simulink model "Bai2_TricycleDrive"  (R2018a)
settings: Solver=VariableStepAuto  StartTime=0.0  StopTime=200  RelTol=1e-3
libraries: simulink x1
settings Model: Creator=Administrator  LastModifiedBy=Administrator

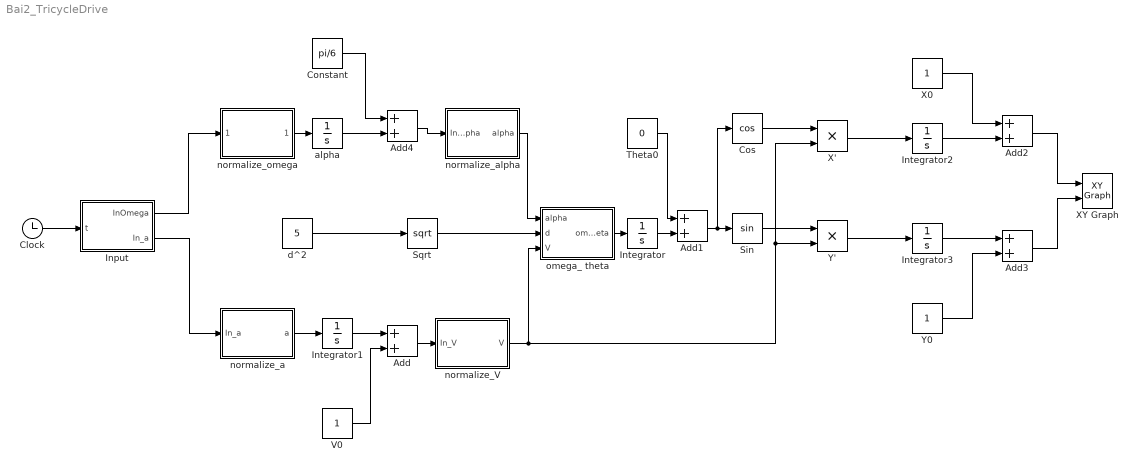
== system Bai2_TricycleDrive ==
  Add{,1..4} (5 alike) : Sum
  Clock : Clock
  Constant : Constant  Value=pi/6
  Cos : Trigonometry  Operator=cos
  Input : MATLAB Function  TreatAsAtomicUnit=on
  Integrator{,1..3} (4 alike) : Integrator
  Sin : Trigonometry
  Sqrt : Sqrt  SaturateOnIntegerOverflow=on
  Theta0 : Constant  Value=0
  V0 : Constant
  X' : Product
  X0 : Constant
  XY Graph : simulink/Sinks/XY Graph  xmin=-10  xmax=10  ymin=0  ymax=20  st=-1
  Y' : Product
  Y0 : Constant
  alpha : Integrator
  d^2 : Constant  Value=5
  normalize_V : MATLAB Function  TreatAsAtomicUnit=on
  normalize_a : MATLAB Function  TreatAsAtomicUnit=on
  normalize_alpha : MATLAB Function  TreatAsAtomicUnit=on
  normalize_omega : MATLAB Function  TreatAsAtomicUnit=on
  omega_ theta : MATLAB Function  TreatAsAtomicUnit=on
  wires:
  Clock/1 -> Input/1(t)
  Input/1(InOmega) -> normalize_omega/1(InOmega)
  Input/2(In_a) -> normalize_a/1(In_a)
  normalize_omega/1(Omega) -> alpha/1
  Add1/1 -> Cos/1, Sin/1
  normalize_a/1(a) -> Integrator1/1
  Integrator1/1 -> Add/1
  Sin/1 -> Y'/1
  Cos/1 -> X'/1
  normalize_V/1(V) -> omega_ theta/3(V), Y'/2, X'/2
  Add/1 -> normalize_V/1(In_V)
  V0/1 -> Add/2
  Theta0/1 -> Add1/1
  X'/1 -> Integrator2/1
  Y'/1 -> Integrator3/1
  Y0/1 -> Add3/2
  Integrator3/1 -> Add3/1
  X0/1 -> Add2/1
  Integrator2/1 -> Add2/2
  Add2/1 -> XY Graph/1
  Add3/1 -> XY Graph/2
  d^2/1 -> Sqrt/1
  Sqrt/1 -> omega_ theta/2(d)
  normalize_alpha/1(alpha) -> omega_ theta/1(alpha)
  Integrator/1 -> Add1/2
  omega_ theta/1(omega_theta) -> Integrator/1
  alpha/1 -> Add4/2
  Add4/1 -> normalize_alpha/1(In_alpha)
  Constant/1 -> Add4/1

== matlab function Bai2_TricycleDrive/normalize_omega ==
  data: InOmega input; Omega output
function Omega = fcn(InOmega)

if(InOmega >= 0.3) Omega = 0.3;
elseif(InOmega <= -0.3) Omega = -0.3;
else Omega = InOmega;
end

== matlab function Bai2_TricycleDrive/Input ==
  data: InOmega output; t input; In_a output
function [InOmega, In_a]= fcn(t)

% a) Van toc va goc lai khong doi
InOmega = 0;
In_a = 0;

% b) Van toc co dinh va goc lai thay doi theo thoi gian
%InOmega = 0.05;
%In_a = 0;

% c) Van toc va goc lai co dinh theo thoi gian
%InOmega = 0.05;
%In_a = 0.1;

== matlab function Bai2_TricycleDrive/normalize_alpha ==
  data: In_alpha input; alpha output
function alpha = fcn(In_alpha)

if(In_alpha >= 3.14/4) alpha = 3.14/4;
elseif(In_alpha <= -3.14/4) alpha = -3.14/4;
else alpha = In_alpha;
end

== matlab function Bai2_TricycleDrive/normalize_a ==
  data: In_a input; a output
function a = fcn(In_a)

if(In_a >= 0.45) a = 0.45;
elseif(In_a <= -0.45) a= -0.45;
else a = In_a;
end

== matlab function Bai2_TricycleDrive/normalize_V ==
  data: In_V input; V output
function V = fcn(In_V)

if(In_V >= 2.25) V = 2.25;
elseif(In_V <= -2.25) V = -2.25;
else V = In_V;
end

== matlab function Bai2_TricycleDrive/omega_ theta ==
  data: alpha input; omega_theta output; d input; V input
function omega_theta = fcn(alpha, d, V)

if(alpha == 0) omega_theta = 0;
else R = d/tan(alpha);
     omega_theta = V / sqrt(d^2 + R^2);
end
